simulink library "vipmisc"  (R2015b)
settings: Solver=ode45  SolverMode=SingleTasking  StartTime=0.0  StopTime=10.0  RelTol=1e-3
undefined symbols (not defined in the file or in its folder): Blocksize
undefined symbols (not defined in the file): Overlapsize
libraries: vipmisc x3
settings Model: ExtModeAutoUpdateStatusClock=off  Creator=The MathWorks, Inc.  LastModifiedBy=The MathWorks, Inc.
settings DataIOCC: SaveFormat=Array  SignalLoggingSaveFormat=ModelDataLogs
settings OptimizationCC: BlockReduction=off  BooleanDataType=off  ExpressionDepthLimit=2147483647
settings DebuggingCC: SaveWithParameterizedLinksMsg=none  UnderspecifiedInitializationDetection=Classic  MergeDetectMultiDrivingBlocksExec=none  SignalResolutionControl=TryResolveAllWithWarning  FcnCallInpInsideContextMsg=UseLocalSettings  StateNameClashWarn=warning  StrictBusMsg=Warning
settings HardwareCC: ProdBitPerPointer=32  ProdLargestAtomicFloat=None  ProdIntDivRoundTo=Undefined  ProdEndianess=Unspecified  ProdWordSize=32  ProdHWDeviceType=32-bit Generic  TargetUnknown=on
settings GRTTargetCC: GeneratePreprocessorConditionals=Disable all  CombineOutputUpdateFcns=off  GRTInterface=on
settings ConfigComp: CovModelRefEnable=Off

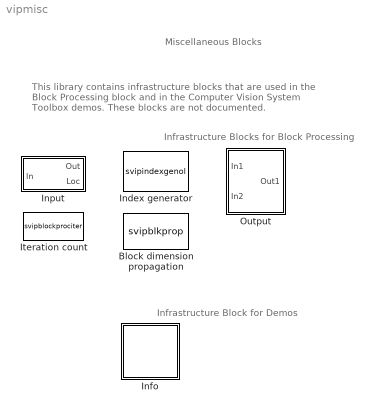
== system vipmisc ==
  note: Miscellaneous Blocks
  note: This library contains infrastructure blocks that are used in
      | the Block Processing block and in the Computer Vision
      | System Toolbox demos.  These blocks are not
      | documented.
  note: Infrastructure Blocks for Block Processing
  note: Infrastructure Block for Demos
  Block dimension propagation : S-Function  FunctionName=svipblkprop  Parameters=szp,oszp  SFunctionDeploymentMode=off  EnableBusSupport=off  mask(Block processing dimension propagation){szp=Blocksize, oszp=Overlapsize}
      mask prompts: szp "Block size:"; oszp "Overlap size:"
      mask help:
      | Propagates correct dimensions to assignment block based on the input size
      | and output size from sub block processing system.
  Index generator : S-Function  FunctionName=svipindexgenol  Parameters=blksize,tverse,ovlpsize,assp,indexst  SFunctionDeploymentMode=off  EnableBusSupport=off  mask(Index generator){blksize=[8 8], ovlpsize=[0 0], tverse=Row-wise, assp=on, indexst=off}
      mask prompts: blksize "Block size:"; ovlpsize "Overlap:"; tverse "Traverse direction:"; assp "Need assign ports"; indexst "Output only start value of index"
      mask help: Index generation for block processing of images.
      mask TypeOptions tverse: Row-wise | Column-wise
      mask Display: disp('Index\ngenerator');
  Info : Subsystem  mask(Info){}
      settings: OpenFcn=web(visiondemohelp, '-helpbrowser');
      mask Display: image('demo_info.bmp','center')
  Input : Subsystem  mask(Input for block processing){Blocksize=Blocksize{1}, Overlapsize=Overlapsize{1}, tverse=Row-wise}
      mask prompts: Blocksize "Block size:"; Overlapsize "Overlap size:"; tverse "Traverse"
      mask TypeOptions tverse: Row-wise | Column-wise
      mask Callback tverse: set_param([gcb '/Index generator'], 'tverse', get_param(gcb, 'tverse'));
  Iteration count : S-Function  FunctionName=svipblockprociter  Parameters=NumI,blksize,ovlpsize  SFunctionDeploymentMode=off  EnableBusSupport=off  mask(Block processing iteration counter){NumI=1, blksize=[2 2], ovlpsize=[0 0]}
      mask prompts: NumI "Number of inputs:"; blksize "Block size:"; ovlpsize "Overlap size:"
      mask help: Finds number of iterations for block processing from the dimensions of the first input and the corresponding block and overlap sizes. Checks if the subsequent inputs are configured to produce the same iteration count.
      mask Display: disp('Iter count');
  Output : Subsystem  mask{Blocksize=Blocksize, Overlapsize=Overlapsize, tverse=Row-wise}
      mask prompts: Blocksize "Block size:"; Overlapsize "Overlap size:"; tverse "Traverse"
      mask TypeOptions tverse: Row-wise | Column-wise
      mask Callback tverse: set_param([gcb '/Index generator'], 'tverse', get_param(gcb, 'tverse'));

== system vipmisc/Info ==

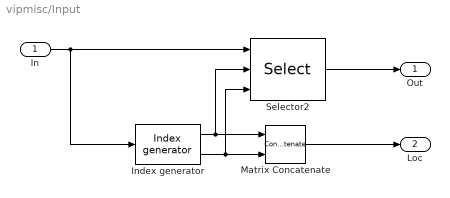
== system vipmisc/Input ==
  In : Inport
  Index generator : vipmisc/Index generator  blksize=Blocksize  ovlpsize=Overlapsize  tverse=Row-wise  assp=off  indexst=on
  Matrix Concatenate : Concatenate  Mode=Multidimensional array
  Selector2 : Selector  NumberOfDimensions=2  IndexMode=Zero-based  InputPortWidth=3  IndexOptions=Starting index (port),Starting index (port)  Indices=1,1  OutputSizes=Blocksize(1),Blocksize(2)
  Out : Outport
  Loc : Outport  Port=2
  wires:
  Selector2/1 -> Out/1
  Index generator/2 -> Selector2/3, Matrix Concatenate/2
  Index generator/1 -> Selector2/2, Matrix Concatenate/1
  In/1 -> Selector2/1, Index generator/1
  Matrix Concatenate/1 -> Loc/1

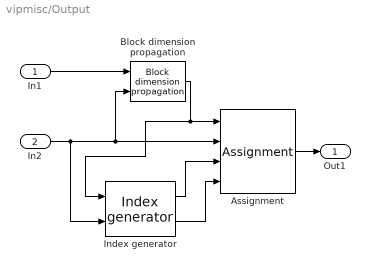
== system vipmisc/Output ==
  In1 : Inport
  In2 : Inport  Port=2
  Assignment : Assignment  NumberOfDimensions=2  IndexMode=Zero-based  DiagnosticForDimensions=Error  IndexOptions=Starting index (port),Starting index (port)  Indices=1,1  OutputSizes=1,1
  Block dimension propagation : vipmisc/Block dimension propagation  szp=Blocksize  oszp=Overlapsize
  Index generator : vipmisc/Index generator  blksize=Blocksize  ovlpsize=Overlapsize  tverse=Row-wise  assp=on  indexst=on
  Out1 : Outport
  wires:
  Block dimension propagation/1 -> Index generator/1, Assignment/1
  In2/1 -> Index generator/2, Block dimension propagation/2, Assignment/2
  In1/1 -> Block dimension propagation/1
  Assignment/1 -> Out1/1
  Index generator/1 -> Assignment/3
  Index generator/2 -> Assignment/4
